simulink model "sps_powersupply_sid"  (R2014a)
settings: Solver=ode23tb  StartTime=0.0  StopTime=0.005  MaxStep=1e-6  RelTol=1e-4
StartFcn:
  | tic;
StopFcn:
  | toc;
libraries: powerlib x17, simulink x1, powerlib_meascontrol x1
Description:
  | Copyright 2008-2012 The MathWorks, Inc.
settings Model: Creator=MathWorks  LastModifiedBy=cosorio
settings DataIOCC: LimitDataPoints=off  SaveOutput=off  SaveTime=off  SignalLoggingName=simoutSPS
settings OptimizationCC: ExpressionDepthLimit=2147483647
settings DebuggingCC: UnderspecifiedInitializationDetection=Classic  FcnCallInpInsideContextMsg=UseLocalSettings  StateNameClashWarn=warning
settings GRTTargetCC: CombineOutputUpdateFcns=off  GRTInterface=on

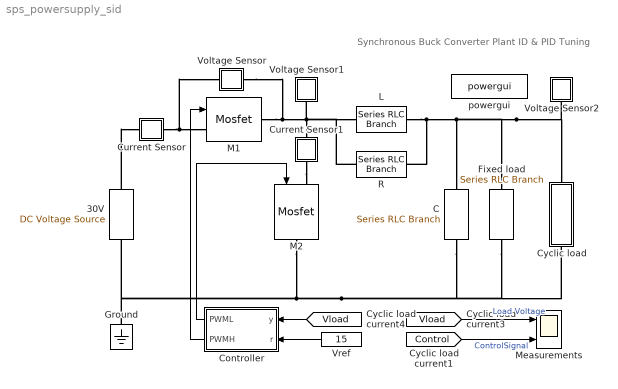
== system sps_powersupply_sid ==
  note: Synchronous Buck Converter
      | Plant ID & PID Tuning
  30V : powerlib/Electrical Sources/DC Voltage Source  Amplitude=30  Measurements=None
  C : powerlib/Elements/Series RLC Branch  LConnTagsString=__new0  RConnTagsString=__new0  BranchType=C  Resistance=1  Inductance=1e-3  SetiL0=off  InitialCurrent=0  Capacitance=22e-6  Setx0=off  InitialVoltage=0  Measurements=None
  Controller : Subsystem
  Current Sensor : Subsystem
      mask Display: disp('i')
  Current Sensor1 : Subsystem
      mask Display: disp('i')
  Cyclic load : Subsystem
  Fixed load : powerlib/Elements/Series RLC Branch  LConnTagsString=__new0  RConnTagsString=__new0  BranchType=R  Resistance=3.75  Inductance=1e-3  SetiL0=off  InitialCurrent=0  Capacitance=1e-6  Setx0=off  InitialVoltage=0  Measurements=None
  Ground : powerlib/Elements/Ground  LConnTagsString=a
  L : powerlib/Elements/Series RLC Branch  LConnTagsString=__new0  RConnTagsString=__new0  BranchType=L  Resistance=15  Inductance=1e-3  SetiL0=off  InitialCurrent=0  Capacitance=1e-6  Setx0=off  InitialVoltage=0  Measurements=None
  M1 : powerlib/Power Electronics/Mosfet  Ron=0.1  Lon=0  Rd=0.01  Vfd=0.8  IC=0  Rs=1e5  Cs=inf  Measurements=off
  M2 : powerlib/Power Electronics/Mosfet  Ron=0.1  Lon=0  Rd=0.01  Vfd=0.8  IC=0  Rs=1e5  Cs=inf  Measurements=off
  Measurements : Scope  NumInputPorts=2
      settings: YMin=0~-0.2  YMax=20~1.2  SaveName=Vload_sps
  R : powerlib/Elements/Series RLC Branch  LConnTagsString=__new0  RConnTagsString=__new0  BranchType=R  Resistance=10e3  Inductance=1e-3  SetiL0=off  InitialCurrent=0  Capacitance=1e-6  Setx0=off  InitialVoltage=0  Measurements=None
  Voltage Sensor : Subsystem
      mask Display: disp('v');
  Voltage Sensor1 : Subsystem
      mask Display: disp('v');
  Voltage Sensor2 : Subsystem
      mask Display: disp('v');
  Vref : Constant  Value=15
  powergui : powerlib/powergui  Priority=1  SimulationMode=Continuous  SolverType=Tustin  SampleTime=1e-7  frequency=60  SPID=off  DisableSnubberDevices=off  DisableRonSwitches=off  DisableVfSwitches=off  SwTol=0  Interpol=off  DisplayEquations=off  Ts=0  methode=off  frequencyindice=0  Pbase=100e6  ErrMax=1e-4  Iterations=50  UnitsV=kV  UnitsW=MW  FunctionMessages=off  echomessages=off  HookPort=off  EnableUseOfTLC=off  x0status=blocks  RestoreLinks=warning  ResistiveCurrentMeasurement=off  Frange=[0:2:500]  Ylog=off  Xlog=on  ShowGrid=off  save=off  variable=ZData  structure=0  ZoomFFT=on  StartTime=0.0  cycles=1  DisplayStyle=1  fundamental=60  FreqAxis=off  MaxFrequency=1000  frequencyindicesteady=1  RmsSteady=1  display=off
  wires:
  Controller/1(PWML) -> M2/1
  Vref/1 -> Controller/2(r)
  [Control] -> Measurements/2  "ControlSignal"
  Controller/2(PWMH) -> M1/1
  [Vload] -> Measurements/1  "Load Voltage"
  [Vload] -> Controller/1(y)
  connections:
  C/RConn1 -- Cyclic load/LConn1 -- Fixed load/RConn1 -- 30V/LConn1 -- Ground/LConn1 -- M2/RConn1
  L/RConn1 -- R/RConn1 -- Cyclic load/RConn1 -- Voltage Sensor2/LConn1 -- Fixed load/LConn1 -- C/LConn1
  M1/RConn1 -- L/LConn1 -- R/LConn1 -- Voltage Sensor1/LConn1 -- Current Sensor1/LConn1 -- Voltage Sensor/RConn1
  30V/RConn1 -- Current Sensor/LConn1
  Current Sensor/RConn1 -- M1/LConn1 -- Voltage Sensor/LConn1
  Current Sensor1/RConn1 -- M2/LConn1

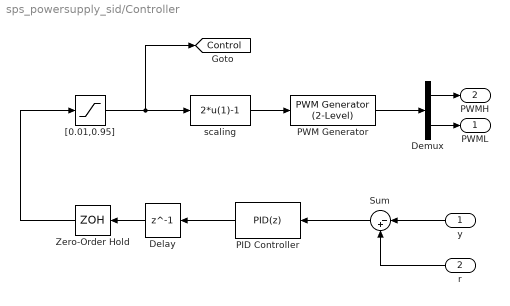
== system sps_powersupply_sid/Controller ==
  y : Inport
  r : Inport  Port=2
  Delay : Delay  DelayLength=1  InputProcessing=Inherited  SampleTime=5e-6
  Demux : Demux  Outputs=2
  PID Controller : simulink/Continuous/PID Controller  Controller=PID  TimeDomain=Discrete-time  SampleTime=5e-6  IntegratorMethod=Forward Euler  FilterMethod=Forward Euler  Form=Parallel  P=1  I=1  D=0  N=100  InitialConditionSource=internal  InitialConditionForIntegrator=0  InitialConditionForFilter=0  ExternalReset=none  LimitOutput=off  UpperSaturationLimit=inf  LowerSaturationLimit=-inf  LinearizeAsGain=on  AntiWindupMode=none  Kb=1  TrackingMode=off  Kt=1  PParamMin=[]  PParamMax=[]  IParamMin=[]  IParamMax=[]  DParamMin=[]  DParamMax=[]  NParamMin=[]  NParamMax=[]  KbParamMin=[]  KbParamMax=[]  KtParamMin=[]  KtParamMax=[]  POutMin=[]  POutMax=[]  IOutMin=[]  IOutMax=[]  DOutMin=[]  DOutMax=[]  NOutMin=[]  NOutMax=[]  KbOutMin=[]  KbOutMax=[]  KtOutMin=[]  KtOutMax=[]  IntegratorOutMin=[]  IntegratorOutMax=[]  FilterOutMin=[]  FilterOutMax=[]  SumOutMin=[]  SumOutMax=[]  SumI1OutMin=[]  SumI1OutMax=[]  SumI2OutMin=[]  SumI2OutMax=[]  SumI3OutMin=[]  SumI3OutMax=[]  SumDOutMin=[]  SumDOutMax=[]  SaturationOutMin=[]  SaturationOutMax=[]  IntegratorContinuousStateAttributes=''  IntegratorStateMustResolveToSignalObject=off  IntegratorRTWStateStorageClass=Auto  FilterContinuousStateAttributes=''  FilterStateMustResolveToSignalObject=off  FilterRTWStateStorageClass=Auto
  PWM Generator : powerlib_meascontrol/Pulse & Signal Generators/PWM Generator (2-Level)  ModulatorType=Single-phase half-bridge (2 pulses)  ModulatorMode=Unsynchronized  nF=27  Fc=50000  ModulatingSignals=off  m=0.8  Freq=60  Phase=0  Ts=0
  Sum : Sum  Inputs=|-+  SaturateOnIntegerOverflow=on  InputSameDT=on  OutDataTypeStr=Inherit: Same as first input
  Zero-Order Hold : ZeroOrderHold  SampleTime=5e-6
  "[0.01,0.95]" : Saturate  UpperLimit=0.95  LowerLimit=.01
  scaling : Fcn  Expr=2*u(1)-1
  PWML : Outport
  PWMH : Outport  Port=2
  tag scope: Control=global
  wires:
  Zero-Order Hold/1 -> "[0.01,0.95]"/1
  y/1 -> Sum/1
  r/1 -> Sum/2
  "[0.01,0.95]"/1 -> scaling/1, [Control]
  scaling/1 -> PWM Generator/1
  Demux/1 -> PWMH/1
  Demux/2 -> PWML/1
  PWM Generator/1 -> Demux/1
  Delay/1 -> Zero-Order Hold/1
  PID Controller/1 -> Delay/1
  Sum/1 -> PID Controller/1

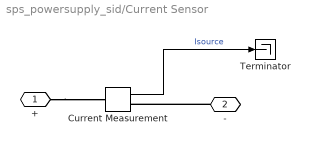
== system sps_powersupply_sid/Current Sensor ==
  Current Measurement : powerlib/Measurements/Current Measurement  PhasorSimulation=off  OutputType=Complex  PSBequivalent=0
  Terminator : Terminator
  + : PMIOPort  Port=1  Side=Left
  - : PMIOPort  Port=2  Side=Right
  wires:
  Current Measurement/1 -> Terminator/1  "Isource"
  connections:
  +/RConn1 -- Current Measurement/LConn1
  -/RConn1 -- Current Measurement/RConn1

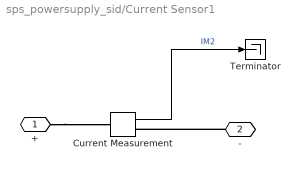
== system sps_powersupply_sid/Current Sensor1 ==
  Current Measurement : powerlib/Measurements/Current Measurement  PhasorSimulation=off  OutputType=Complex  PSBequivalent=0
  Terminator : Terminator
  + : PMIOPort  Port=1  Side=Left
  - : PMIOPort  Port=2  Side=Right
  wires:
  Current Measurement/1 -> Terminator/1  "IM2"
  connections:
  -/RConn1 -- Current Measurement/RConn1
  +/RConn1 -- Current Measurement/LConn1

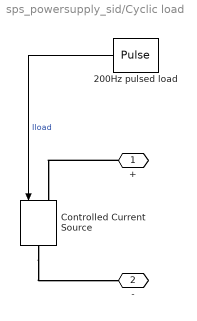
== system sps_powersupply_sid/Cyclic load ==
  200Hz pulsed load : DiscretePulseGenerator  PulseType=Time based  Amplitude=2  Period=1/200  PulseWidth=50  PhaseDelay=1/400
  Controlled Current Source : powerlib/Electrical Sources/Controlled Current Source  Initialize=on  Source_Type=AC  Amplitude=0  Phase=0  Frequency=0  Measurements=None
  + : PMIOPort  Port=1  Side=Right
  - : PMIOPort  Port=2  Side=Left
  wires:
  200Hz pulsed load/1 -> Controlled Current Source/1  "Iload"
  connections:
  Controlled Current Source/RConn1 -- -/RConn1
  +/RConn1 -- Controlled Current Source/LConn1

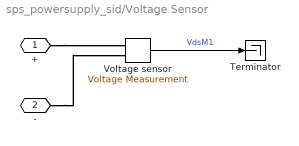
== system sps_powersupply_sid/Voltage Sensor ==
  Terminator : Terminator
  Voltage sensor : powerlib/Measurements/Voltage Measurement  PhasorSimulation=off  OutputType=Complex  PSBequivalent=0
  + : PMIOPort  Port=1  Side=Left
  - : PMIOPort  Port=2  Side=Right
  wires:
  Voltage sensor/1 -> Terminator/1  "VdsM1"
  connections:
  +/RConn1 -- Voltage sensor/LConn1
  -/RConn1 -- Voltage sensor/LConn2

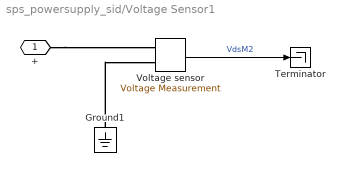
== system sps_powersupply_sid/Voltage Sensor1 ==
  Ground1 : powerlib/Elements/Ground  LConnTagsString=a
  Terminator : Terminator
  Voltage sensor : powerlib/Measurements/Voltage Measurement  PhasorSimulation=off  OutputType=Complex  PSBequivalent=0
  + : PMIOPort  Port=1  Side=Left
  wires:
  Voltage sensor/1 -> Terminator/1  "VdsM2"
  connections:
  Ground1/LConn1 -- Voltage sensor/LConn2
  +/RConn1 -- Voltage sensor/LConn1

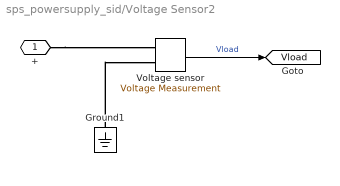
== system sps_powersupply_sid/Voltage Sensor2 ==
  Ground1 : powerlib/Elements/Ground  LConnTagsString=a
  Voltage sensor : powerlib/Measurements/Voltage Measurement  PhasorSimulation=off  OutputType=Complex  PSBequivalent=0
  + : PMIOPort  Port=1  Side=Left
  tag scope: Vload=global
  wires:
  Voltage sensor/1 -> [Vload]  "Vload"
  connections:
  +/RConn1 -- Voltage sensor/LConn1
  Ground1/LConn1 -- Voltage sensor/LConn2
